simulink library "Lib_EMTAT"  (R2021b)
settings: Solver=VariableStepAuto  StartTime=0.0  StopTime=10.0  RelTol=1e-3
undefined symbols (not defined in the file or in its folder): A_M, B_M, Cj, component_degradation_input, Cs, E0_M, f_sw, K_M, MWS, Q_M, Q_rr, r_c, r_D, R_M, Rj, Ru, SNR_DX_M, SNR_IC_M, SNR_Mn_M, SNR_Mx_M, SOC_Init_M, u_ce0, u_D0
libraries: $bdroot x82, simulink x23, Lib_Dyn_StateSpace_EMTAT x3, PB_Library_Master_Working x1
(part 1 of 7)
settings Model: Creator=sbianco1  LastModifiedBy=sbianco1
settings SolverCC: AlgebraicLoopSolver=TrustRegion
settings OptimizationCC: BlockReduction=off  DefaultParameterBehavior=Inlined  BufferReuse=off
settings DebuggingCC: SFMachineParentedDataDiag=warning

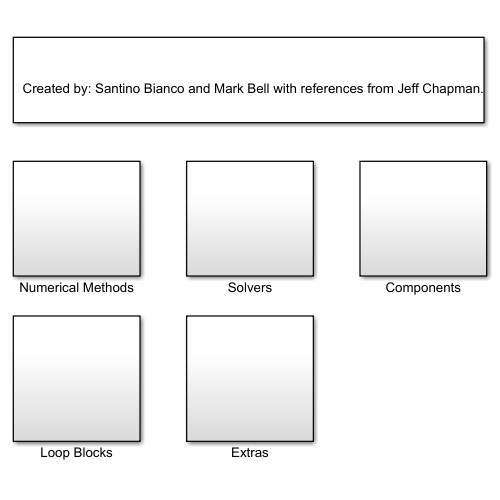
[thumbnail: Simulink's stored preview of the top-level diagram]
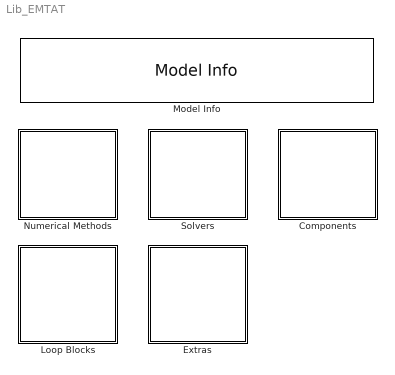
== system Lib_EMTAT ==
  Components : Subsystem
  Extras : Subsystem
  Loop Blocks : Subsystem
  Model Info : simulink/Model-Wide Utilities/Model Info  Frame=on  DisplayStringWithTags=Created by: Santino Bianco and Mark Bell with references from Jeff Chapman.  HorizontalTextAlignment=Left  LeftAlignmentValue=0.02
  Numerical Methods : Subsystem
  Solvers : Subsystem

== system Lib_EMTAT/Components ==
  Physics-Based : Subsystem
  Power Flow : Subsystem

== system Lib_EMTAT/Extras ==
  Exergy (Heat) : Subsystem  mask(Exergy){m=0, Cp=0}
      mask prompts: m "m - Mass, slug"; Cp "Cp - Specific Heat, Btu/slug-degF"
      mask help: This block calculated the exergy of a component given the component's generated heat, mass, material specific heat, and chnage in ambient temperature from sea level static (SLS).
      settings: AttributesFormatString=|
      | Exergy
      | Version: %<LibraryVersion>
  Exergy (Ploss) : Subsystem  mask(Exergy){m=0, Cp=0, Qo=0}
      mask prompts: m "m - Mass, slug"; Cp "Cp - Specific Heat, Btu/slug-degF"; Qo "Qo - Initial Heat, Btu"
      mask help: This block calculated the exergy of a component given the component's generated heat, mass, material specific heat, and chnage in ambient temperature from sea level static (SLS).
      settings: AttributesFormatString=|
      | Exergy
      | Version: %<LibraryVersion>
  Temperature (Heat) : Subsystem  mask(Temperature){m=0, Cp=0}
      mask prompts: m "m - Mass, lbm"; Cp "Cp - Specific Heat, Btu/(lbm-degF)"
      mask help: This block converts a heat output (Heat) from an electrical component to a temperature (Temp) using the ambient temperature (Ambient Temp) and possibly a change in ambient temperature from sea-level static (dTamb) as inputs. A mass in units of pound-mass and a specific heat in units of Btu/(lbm-degF) must be specified.
      settings: AttributesFormatString=|
      | Temperature
      | Version: %<LibraryVersion>
      mask DialogControl Container3 Prompt: Physical Parameters
  Temperature (Ploss) : Subsystem  mask(Temperature){m=0, Cp=0, Qo=0}
      mask prompts: m "m - Mass, lbm"; Cp "Cp - Specific Heat, Btu/(lbm-degF)"; Qo "Qo - Initial Heat, Btu"
      mask help: This block converts a heat output (Heat) from an electrical component to a temperature (Temp) using the ambient temperature (Ambient Temp) and possibly a change in ambient temperature from sea-level static (dTamb) as inputs. A mass in units of pound-mass and a specific heat in units of Btu/(lbm-degF) must be specified.
      settings: AttributesFormatString=|
      | Temperature
      | Version: %<LibraryVersion>
      mask DialogControl Container3 Prompt: Physical Parameters

== system Lib_EMTAT/Loop Blocks ==
  Outer Loop Integrator : Subsystem  mask(Outer Loop Integrator){Xo=0}
      mask prompts: Xo "Xo - Initial State Conditions"
      mask help: The Outer Loop Integrator takes in a vector of state variables and integrates each variable using a Continuous Integrator block.
      settings: AttributesFormatString=|
      | Outer Loop Integrator
      | Version: %<LibraryVersion>
      mask DialogControl fsfd Prompt: Parameters
  Outer Loop Time Step Delay : Subsystem  mask(Outer Loop Time Step Delay){Wo=0}
      mask prompts: Wo "Wo - Initial Conditions"
      mask help: The Outer Loop Time Step Delay block takes in a vector of variables and applies a one time step delay to each variable in the vector using a Unit Delay block.
      settings: AttributesFormatString=|
      | OuterLoop Time Step Delay
      | Version: %<LibraryVersion>
      mask DialogControl fsdf Prompt: Parameters

== system Lib_EMTAT/Numerical Methods ==
  Jacobian Calculator : Subsystem  TreatAsAtomicUnit=on  mask(T-MATS: Jacobian Calculator Library Block){N_Per_M=[0.01 0.01 0.01;-0.01 -0.01 -0.01]}
      mask prompts: N_Per_M "N_Per_M - Perturbations (nxm)"
      mask help:
      | The Jacobian Calculator block calculates the Jabobian of the system by perturbing the system around an initial point and calculating the gradient for each perturbation. This module will run once on start up and then again only if the reset is pressed.
      | Below: n (rows) is the number of times each independent will be perturbed and m (columns) is the number of inputs.
      settings: AttributesFormatString=|
      | Jacobian Calculator
      | Version: %<LibraryVersion>
      mask Help: web(which('NumMthd_TMATS_JC.html'),'-helpbrowser')
  Newton Raphson Solver : Subsystem  TreatAsAtomicUnit=on  mask(T-MATS: Newton Raphson Solver Library Block){NR_IC_M=SNR_IC_M./abs(SNR_IC_M), NR_dx_Lim_M=SNR_DX_M, NR_Mx_Lim_M=SNR_Mx_M./abs(SNR_IC_M), NR_Mn_Lim_M=SNR_Mn_M./abs(SNR_IC_M), BlkNm_M=double(gcb)}
      mask prompts: NR_IC_M "NR_IC_M - Initial Conditions of Newton Raphson (mx1)"; NR_dx_Lim_M "NR_dx_Lim_M - Newton Raphson step size limit (%) (1x1)"; NR_Mx_Lim_M "NR_Mx_Lim_M - Max limit (1x1 or mx1)"; NR_Mn_Lim_M "NR_Mn_Lim_M - Min Limit (1x1 or mx1)"; BlkNm_M "BlkNm_M - Block Name"
      mask help:
      | Newton Raphson Solver:
      |
      | x(n+1) = x(n) - inverse(f'(x(n)))*f(x(n))
      |
      | Note:
      | inverse(f'(x(n))) is an m x m matrix and f(x(n)) is an m x 1 matrix
      | where m is the length of the initial conditions matrix and number of system independents.
      mask init:
      | if isequal(size(NR_Mx_Lim_M),size(NR_IC_M))
      | elseif isequal(size(NR_Mx_Lim_M),size(1))
      | else
      |     warning('NR_Mx_Lim_M must be the same size as NR_IC_M or a constant')
      | end
      | 
      | if isequal(size(NR_Mn_Lim_M),size(NR_IC_M))
      | elseif isequal(size(NR_Mn_Lim_M),size(1))
      | else
      |     warning('NR_Mn_Lim_M must be the same size as NR_IC_M or a constant')
      | end
      settings: AttributesFormatString=|
      | Newton Raphson Solver
      | Verson: %<LibraryVersion>
      mask Help: web(which('NumMthd_TMATS_NRS.html'),'-helpbrowser')

== system Lib_EMTAT/Solvers ==
  Iterative NR Solver w JacobianCalc : Subsystem  mask(T-MATS: Iterative NR Solver w Jacobian Calc Library Block){SJac_Per_M=[0.01 0.01 0.01;-0.01 -0.01 -0.01], SNR_IC_M=[1; 2; 3], SNR_DX_M=5, SNR_Mx_M=100000, SNR_Mn_M=0.0001, SJacobianAttempts_M=20, Cond_Limits_M=0.0001}
      mask prompts: SJac_Per_M "SJac_Per_M - Jacobian Perturbation size (frac) (nxm)"; SNR_IC_M "SNR_IC_M - Newton Raphson Initial Conditions (mx1)"; SNR_DX_M "SNR_DX_M - Newton Raphson step size limiter (%) (1x1)"; SNR_Mx_M "SNR_Mx_M - Newton Raphson max limit (1x1 or mx1)"; SNR_Mn_M "SNR_Mn_M - Newton Raphson min limit (1x1 or mx1)"; SJacobianAttempts_M "SJacobianAttempts_M - Newton Raphson attempts before the Jacobian recalculation (1x1)"; Cond_Limits_M "Cond_Limits_M - Iteration Conditions Limits (mx1 or 1x1)"
      mask help:
      | The Iterative Newton Raphson Solver with Jacobian Calculator block will
      | supply the inputs to iteratively drive the outputs of a system to zero.
      |
      | This will be performed in three steps.
      | 1) Jabobian calculator sends Perturbations to the plant then calculates the plant
      | Jacboian based on the system response
      | 2) The Newton Raphson will use the inverse of the Jacobian to iteratively step the
      | system toward solution.
      | 3) Once the solution has satisfied the conditions the Newton Raphson is shut off.
      |
      | This module is designed for dynamic systems and should be paired with
      | a "do... while" block in Simulink. The "do...while" block and this module
      | should both be located in the same subsystem as the plant that is to be solved for.
      mask init:
      | if isequal(size(SNR_Mx_M),size(SNR_IC_M))
      | elseif isequal(size(SNR_Mx_M),[1 1])
      | else
      |     disp('NR_Mx_Lim_M must be the same size as NR_IC_M or a constant')
      | end
      | 
      | if isequal(size(SNR_Mn_M),size(SNR_IC_M))
      | elseif isequal(size(SNR_Mn_M),[1 1])
      | else
      |     disp('NR_Mn_Lim_M must be the same size as NR_IC_M or a constant')
      | end
      settings: AttributesFormatString=|
      | Iterative NR Solver w JacobianCalc
      | Version: %<LibraryVersion>
      mask Help: web(which('Solver_TMATS_INRSwJC.html'),'-helpbrowser')
  "SS NR Solver w JacobianCalc " : Subsystem  mask(T-MATS: SS NR Solver w Jacobian Calc Library Block){SJac_Per_M=[0.01 0.01 0.01;-0.01 -0.01,-0.01], SNR_IC_M=[1; 2; 3], SNR_DX_M=5, SNR_Mx_M=100000, SNR_Mn_M=0.00001, SJacobianAttempts_M=20, Cond_Limits_M=0.0001}
      mask prompts: SJac_Per_M "SJac_Per_M - Jacobian Perturbation size (frac)(nxm)"; SNR_IC_M "SNR_IC_M - Newton Raphson Initial Conditions (mx1)"; SNR_DX_M "SNR_DX_M - Newton Raphson step size limit (%) (1x1)"; SNR_Mx_M "SNR_Mx_M - Newton Raphson max limit (1x1 or mx1)"; SNR_Mn_M "SNR_Mn_M - Newton Raphson min limit (1x1 or mx1)"; SJacobianAttempts_M "SJacobianAttempts_M - Newton Raphson attempts before the Jacobian recalculation (1x1)"; Cond_Limits_M "Cond_Limits_M - Iteration Conditions Limits (mx1 or 1x1)"
      mask help:
      | The Steady State Newton Raphson Solver with Jacobian Calculator block will
      | supply the inputs to iteratively drive the outputs of a system to zero.
      |
      | This will be performed in three steps.
      | 1) Jabobian calculator sends Perturbations to the plant then calculates the plant
      | Jacboian based on the system response
      | 2) The Newton Raphson will use the inverse of the Jacobian to iteratively step the
      | system toward solution.
      | 3) Once the solution has satisfied the conditions the Newton Raphson is shut off.
      |
      | Simulation run time length should be selected as to give the Newton Raphson solver adequate time to develop a solution.
      mask init: same as Lib_EMTAT/Solvers/Iterative NR Solver w JacobianCalc
      settings: AttributesFormatString=|
      | SS NR Solver w JacobianCalc
      | Version: %<LibraryVersion>
      mask Help: web(which('Solver_TMATS_SSNRwJC.html'),'-helpbrowser')
